simulink model "c"  (R2024b)
settings: Solver=VariableStepAuto  StartTime=0.0  StopTime=18000  RelTol=1e-3
undefined symbols (not defined in the file): Ion, Lithium
libraries: simulink x2, spsBatteryLib x1, spsSeriesRLCBranchLib x1, SignalEditorBlockLib x1, sps_lib x1
settings Model: Creator=lenovo  LastModifiedBy=lenovo

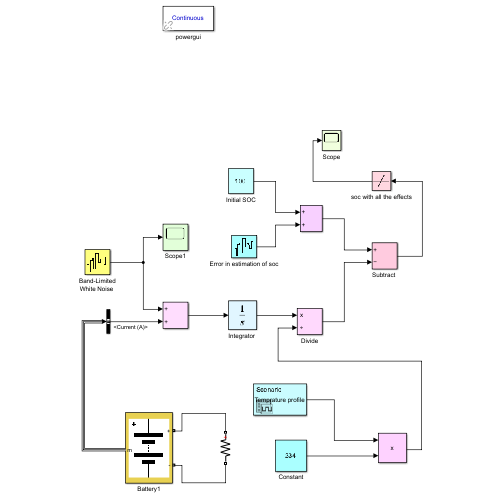
[thumbnail: Simulink's stored preview of the top-level diagram]
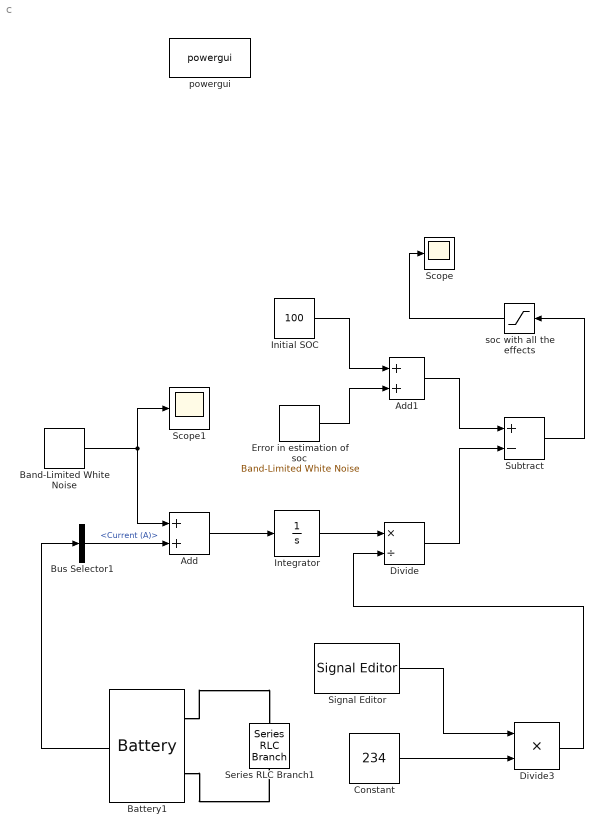
== system c ==
  Add : Sum
  Add1 : Sum
  "Band-Limited White Noise " : simulink/Sources/Band-Limited White Noise  Cov=[0.1]  Ts=0.1  seed=[23341]
  Battery1 : spsBatteryLib/Battery  BatType=Lithium-Ion  NomV=1.18  NomQ=6.5  SOC=100  Batt_Tr=0  PresetModel=on  MaxQ=6.5  MinV=0.885  FullV=1.3735  Dis_rate=2.8261  R=0.0018154  Normal_OP=5.8783  expZone="[1.2749     0.31935]"
  Bus Selector1 : BusSelector  OutputSignals=Current (A)
  Constant : Constant  Value=234
  Divide : Product  Inputs=*/
  Divide3 : Product  Inputs=**
  Error in estimation of soc : simulink/Sources/Band-Limited White Noise  Cov=[0.1]  Ts=0.1  seed=[23341]
  Initial SOC : Constant  Value=100
  "Integrator " : Integrator
  Scope : Scope
  Scope1 : Scope
  Series RLC Branch1 : spsSeriesRLCBranchLib/Series RLC Branch  LConnTagsString=__new0  RConnTagsString=__new0  BranchType=R  Resistance=.5  Inductance=0  SetiL0=off  InitialCurrent=0  Capacitance=0  Setx0=off  InitialVoltage=0  Measurements=None
  Signal Editor : SignalEditorBlockLib/Signal Editor  FileName=Temp profile.mat  ActiveScenario=Scenario  ActiveSignal=Temprature profile  IsBus=off  OutputBusObjectStr=Bus: BusObject  SampleTime=0  Interpolate=off  ZeroCross=off  OutputAfterFinalValue=Setting to zero  Unit=inherit  PreserveSignalName=on  ApplySigPropsToAllScenarios=on  ApplySigPropsToAllSignals=off
  "Subtract " : Sum  Inputs=+-
  powergui : sps_lib/powergui  Priority=1  SimulationMode=Continuous  SampleTime=50e-6  frequency=60  Iterations=50  frequencyindice=0  Pbase=100e6  ErrMax=1e-4  UnitsV=kV  UnitsW=MW  buscounter=0  FunctionMessages=off  echomessages=off  EnableUseOfTLC=off  CurrentSourceSwitches=off  DisableSnubberDevices=off  DisableRonSwitches=off  DisableVfSwitches=off  DisplayEquations=off  AutomaticDiscreteSolvers=off  SolverType=Tustin/Backward Euler (TBE)  Interpol=off  ExternalGateDelay=off  methode=off  Ts=100  x0status=blocks  SPID=on  SwTol=0  HookPort=off  NonlinearTolerance=1e-4  nMaxIteration=100  ContinueOnMaxIteration=off  RestoreLinks=warning  ResistiveCurrentMeasurement=off  Frange=[0:2:500]  Ylog=off  Xlog=on  ShowGrid=off  save=off  variable=ZData  structure=0  ZoomFFT=off  StartTime=0.0  cycles=1  DisplayStyle=1  fundamental=60  FreqAxis=off  MaxFrequency=1000  frequencyindicesteady=1  RmsSteady=1  display=off
  soc with all the effects : Saturate  UpperLimit=150  LowerLimit=0
  wires:
  "Band-Limited White Noise "/1 -> Scope1/1, Add/1
  soc with all the effects/1 -> Scope/1
  Divide3/1 -> Divide/2
  Divide/1 -> "Subtract "/2
  "Integrator "/1 -> Divide/1
  Signal Editor/1 -> Divide3/1
  Bus Selector1/1 -> Add/2  "<Current (A)>"
  Battery1/1 -> Bus Selector1/1
  Add/1 -> "Integrator "/1
  "Subtract "/1 -> soc with all the effects/1
  Constant/1 -> Divide3/2
  Initial SOC/1 -> Add1/1
  Error in estimation of soc/1 -> Add1/2
  Add1/1 -> "Subtract "/1
  connections:
  Battery1/LConn2 -- Series RLC Branch1/RConn1
  Battery1/LConn1 -- Series RLC Branch1/LConn1
